simulink model "single_phase_grid_connected_inverter"  (R2022b)
settings: Solver=FixedStepDiscrete  StartTime=0.0  StopTime=0.5  FixedStep=1e-6  RelTol=1e-3
libraries: spsSeriesRLCBranchLib x9, spsFourierLib x8, spsMosfetLib x4, spsCurrentMeasurementLib x3, simulink x3, spsVoltageMeasurementLib x3, spsMeanLib x2, spsRMSLib x2, spsDCVoltageSourceLib x1, spsIdealSwitchLib x1, spspowerguiLib x1, spsControlledVoltageSourceLib x1
(part 2 of 2)

== matlab function single_phase_grid_connected_inverter/MATLAB Function20 ==
  data: u_alpha input; theta output; u_beta input; qerror output
function [theta, qerror] = SRF_PLL(u_alpha, u_beta)
% 同步旋转坐标系锁相环 SRF-PLL
% 【已修改为：纯自适应频率版本 → 和你主循环PLL完全一致】
% 输入：u_alpha, u_beta
% 输出：theta 锁相相位, qerror q分量（趋近0）

    %% ===================== 1. 固定参数 =====================
    Ts = 5e-5;               % 20kHz 采样步长（必须匹配）
    
    % PI参数（和你主循环一致）
    kp_pll = 200;
    ki_pll = 7000;

    %% ===================== 2. 持久变量 =====================
    persistent theta_prev
    persistent integral_pll
    
    if isempty(theta_prev)
        theta_prev = 0;
        integral_pll = 0;
    end

    %% ===================== 3. Park 变换 =====================
    cos_theta = cos(theta_prev);
    sin_theta = sin(theta_prev);
    
    u_d =  u_alpha * cos_theta + u_beta * sin_theta;
    u_q = -u_alpha * sin_theta + u_beta * cos_theta;
    
    qerror = u_q;  % q分量（锁相成功→0）

    %% ===================== 4. PI控制器（我的版本：直接输出ω） =====================
    integral_pll = integral_pll + qerror * Ts;          % 积分
    omega_pll    = kp_pll * qerror + ki_pll * integral_pll; % 直接输出角频率

    %% ===================== 5. 积分生成相位 =====================
    theta = theta_prev + omega_pll * Ts;

    %% ===================== 6. 相位归一化（±π） =====================
    if theta > pi
        theta = theta - 2*pi;
    elseif theta < -pi
        theta = theta + 2*pi;
    end

    %% ===================== 7. 更新状态 =====================
    theta_prev = theta;
end

== matlab function single_phase_grid_connected_inverter/级联谐波抑制4 ==
  data: u input; y output
function y = Cascade_Notch_Filter(u)
% 级联陷波滤波器：滤除3/5/7次固定频率谐波（150/250/350Hz）
% 输入u：待滤波的标量信号
% 输出y：滤波后的标量信号
% 适配：20kHz采样率（Ts=5e-5），和你的控制环完全对齐

    persistent x3_1 x3_2 x5_1 x5_2 x7_1 x7_2 first_run
    persistent b3_0 b3_1 b3_2 a3_1 a3_2
    persistent b5_0 b5_1 b5_2 a5_1 a5_2
    persistent b7_0 b7_1 b7_2 a7_1 a7_2

    %% ===================== 1. 初始化：仅首次运行 =====================
    if isempty(first_run)
        % --- 固定参数 ---
        Fs = 2e4;          % 采样频率 20kHz
        Ts = 1/Fs;            % 采样周期 5e-5s
        wc = 10;              % 截止角频率 25 rad/s
        
        % 目标谐波频率
        w3 = 2*pi*150;  % 3次谐波 150Hz
        w5 = 2*pi*250;  % 5次谐波 250Hz
        w7 = 2*pi*350;  % 7次谐波 350Hz

        % --- Tustin变换预计算系数 ---
        k = 2/Ts;
        k2 = k*k;

        % --- 3次滤波器系数 ---
        [b3_0, b3_1, b3_2, a3_1, a3_2] = calc_coeff(w3, wc, k, k2);
        % --- 5次滤波器系数 ---
        [b5_0, b5_1, b5_2, a5_1, a5_2] = calc_coeff(w5, wc, k, k2);
        % --- 7次滤波器系数 ---
        [b7_0, b7_1, b7_2, a7_1, a7_2] = calc_coeff(w7, wc, k, k2);

        % --- 显式初始化状态变量为标量 ---
        x3_1 = 0; x3_2 = 0;
        x5_1 = 0; x5_2 = 0;
        x7_1 = 0; x7_2 = 0;
        
        first_run = 1;
    end

    %% ===================== 2. 级联滤波计算（显式差分方程） =====================
    % --- 第1级：3次谐波滤波 ---
    y3 = b3_0*u + x3_1;
    x3_1_next = b3_1*u - a3_1*y3 + x3_2;
    x3_2_next = b3_2*u - a3_2*y3;
    
    % --- 第2级：5次谐波滤波 ---
    y5 = b5_0*y3 + x5_1;
    x5_1_next = b5_1*y3 - a5_1*y5 + x5_2;
    x5_2_next = b5_2*y3 - a5_2*y5;
    
    % --- 第3级：7次谐波滤波 ---
    y7 = b7_0*y5 + x7_1;
    x7_1_next = b7_1*y5 - a7_1*y7 + x7_2;
    x7_2_next = b7_2*y5 - a7_2*y7;
    
    % --- 更新状态变量 ---
    x3_1 = x3_1_next; x3_2 = x3_2_next;
    x5_1 = x5_1_next; x5_2 = x5_2_next;
    x7_1 = x7_1_next; x7_2 = x7_2_next;
    
    % --- 最终输出 ---
    y = y7;

end

%% ===================== 局部函数：预计算滤波器系数 =====================
function [b0, b1, b2, a1, a2] = calc_coeff(wn, wc, k, k2)
    % 连续域：G(s) = (s^2 + wn^2) / (s^2 + 2*wc*s + wn^2)
    % Tustin离散化：s = k*(z-1)/(z+1)
    
    % 连续域系数
    num_b0 = 1; num_b1 = 0; num_b2 = wn^2;
    den_a0 = 1; den_a1 = 2*wc; den_a2 = wn^2;
    
    % 离散化计算
    B0 = num_b0*k2 + num_b1*k + num_b2;
    B1 = 2*num_b2 - 2*num_b0*k2;
    B2 = num_b0*k2 - num_b1*k + num_b2;
    
    A0 = den_a0*k2 + den_a1*k + den_a2;
    A1 = 2*den_a2 - 2*den_a0*k2;
    A2 = den_a0*k2 - den_a1*k + den_a2;
    
    % 归一化（a0=1）
    b0 = B0 / A0;
    b1 = B1 / A0;
    b2 = B2 / A0;
    a1 = A1 / A0;
    a2 = A2 / A0;
end

== matlab function single_phase_grid_connected_inverter/MATLAB Function11 ==
  data: u_alpha input; theta output; u_beta input; qerror output
function [theta, qerror] = SRF_PLL(u_alpha, u_beta)
% 同步旋转坐标系锁相环 SRF-PLL（严格匹配框图逻辑）
% 输入
%   u_alpha:  α轴输入信号（对应框图的v'，与电网电压同相）
%   u_beta:   β轴输入信号（对应框图的qv'，与电网电压正交90°）
% 输出
%   theta:    锁相得到的电网相位 [0, 2π)
%   qerror:   q轴相位误差（锁相锁定时趋近于0）
% 适配：仿真步长 Ts=1e-5（10kHz采样），基波频率50Hz

    %% ===================== 1. 固定参数配置 =====================
    Ts = 1e-5;               % 采样时间，必须与全局仿真步长完全一致
    f0 = 50;                  % 电网额定基波频率 (Hz)
    w0 = 2 * pi * f0;        % 额定角频率 (rad/s)
    
    % PI控制器参数（适配10kHz采样，可按需调整）
    kp_pll = 60;              % 比例系数：增大加快锁相响应，过大易振荡
    ki_pll = 5000;            % 积分系数：增大减小稳态相位误差，过大影响稳定性

    %% ===================== 2. 持久变量初始化（仅首次运行执行） =====================
    persistent theta_prev     % 上一拍的锁相相位
    persistent xi_pll         % PI控制器的积分项（抗饱和）
    
    if isempty(theta_prev)
        theta_prev = 0;       % 相位初始值清零
        xi_pll = 0;           % 积分项初始值清零
    end

    %% ===================== 3. αβ/dq 帕克变换（核心鉴相环节） =====================
    % 标准帕克变换矩阵，严格匹配框图逻辑
    % [u_d]   = [ cosθ   sinθ ] [u_alpha]
    % [u_q]     [ -sinθ  cosθ ] [u_beta ]
    cos_theta = cos(theta_prev);
    sin_theta = sin(theta_prev);
    
    u_d = u_alpha * cos_theta + u_beta * sin_theta;  % d轴分量（对应电压幅值）
    u_q = -u_alpha * sin_theta + u_beta * cos_theta; % q轴分量（相位误差）
    
    qerror = u_q; % 输出q轴相位误差，锁相锁定时qerror→0

    %% ===================== 4. PI环路控制器 =====================
    % 位置式PI控制器，带积分抗饱和
    xi_pll = xi_pll + ki_pll * Ts * qerror;  % 积分项更新
    delta_w = kp_pll * qerror + xi_pll;      % 频率偏差量
    w_pll = w0 + delta_w;                     % 锁相得到的实时角频率

    %% ===================== 5. 积分环节（1/s）生成相位 =====================
    % 前向欧拉离散化，对应框图的1/s积分环节
    theta = theta_prev + Ts * w_pll;
    
    % 相位归一化到 [0, 2π)，防止数值溢出
    theta = mod(theta, 2 * pi);

    %% ===================== 6. 更新状态变量（为下一拍迭代准备） =====================
    theta_prev = theta;

end

== matlab function single_phase_grid_connected_inverter/MATLAB Function2 ==
  data: u input; y output
function y = SecondOrderPadeDelay_1p5Ts(u)
% 二阶Padé逼近1.5Ts延迟模块（直接从闭环仿真提取，已验证直流增益=1）
% 输入：u - 待延迟的信号（如PR控制器输出）
% 输出：y - 延迟后的信号
% 适配：与你的闭环仿真参数100%匹配，直流增益严格等于1

persistent u_prev1 u_prev2 y_prev1 y_prev2 first_run

%% 初始化：仅首次运行
if isempty(first_run)
    % 初始化状态变量（二阶需要2个历史输入+2个历史输出）
    u_prev1 = 0;
    u_prev2 = 0;
    y_prev1 = 0;
    y_prev2 = 0;
    
    first_run = true;
end

%% 【核心】直接从闭环仿真提取的系数（已验证直流增益=1）
b0 = 0.076923076923077;
b1 = 0.153846153846154;
b2 = 1.000000000000000;
a1 = -0.153846153846154;
a2 = -0.076923076923077;

%% 二阶离散差分方程计算延迟输出
y = b0*u + b1*u_prev1 + b2*u_prev2 ...
    + a1*y_prev1 + a2*y_prev2;

%% 更新状态变量（供下一时刻使用）
u_prev2 = u_prev1;
u_prev1 = u;
y_prev2 = y_prev1;
y_prev1 = y;
end

== matlab function single_phase_grid_connected_inverter/MATLAB Function3 ==
  settings: updateMethod=DISCRETE
  data: u input; y output
function y = PR_Controller(u)
% 准谐振PR控制器，和你的.m文件1:1完全匹配
% 输入u：误差信号 error = Iref - iL2
% 输出y：PR控制器输出的调制波

persistent x_prev1 x_prev2 y_prev1 y_prev2 first_run

%% 1. 固定参数（和.m文件完全一致，无任何修改）
Ts = 5e-5;           % 采样时间 (s)，20kHz控制环
Kp = 0.254;          % PR比例系数
Kr = 50;             % PR谐振系数
w0 = 2*pi*50;        % 基波角频率 (50Hz)，和.m文件写法完全对齐
wi = pi;             % PR谐振带宽

%% 2. 初始化状态变量（仅首次运行，和.m文件初始值一致）
if isempty(first_run)
    x_prev1 = 0;  % 对应.m文件的x1_pr：上一时刻的误差
    x_prev2 = 0;  % 对应.m文件的x2_pr：上两时刻的误差
    y_prev1 = 0;  % 对应.m文件的y1_pr：上一时刻的输出
    y_prev2 = 0;  % 对应.m文件的y2_pr：上两时刻的输出
    first_run = true;
end

%% 3. 离散化系数计算（和.m文件公式、参数完全一致）
a0_pr = 4 + 2*wi*Ts + w0^2*Ts^2;
a1_pr = 2*w0^2*Ts^2 - 8;
a2_pr = 4 - 2*wi*Ts + w0^2*Ts^2;

b0_pr = 4*Kp + 4*Kp*wi*Ts + 4*Kr*wi*Ts + Kp*w0^2*Ts^2;
b1_pr = 2*Kp*w0^2*Ts^2 - 8*Kp;
b2_pr = 4*Kp - 4*Kp*wi*Ts - 4*Kr*wi*Ts + Kp*w0^2*Ts^2;

%% 4. 差分方程计算输出（和.m文件公式完全一致，符号无错误）
y = (b0_pr*u + b1_pr*x_prev1 + b2_pr*x_prev2 ...
    - a1_pr*y_prev1 - a2_pr*y_prev2) / a0_pr;

%% 5. 输出限幅（和.m文件完全一致，[-1,1]）
MODULATION_MAX = 1;
MODULATION_MIN = -1;
y = max(min(y, MODULATION_MAX), MODULATION_MIN);

%% 6. 更新状态变量（和.m文件执行顺序完全一致：先算输出→再限幅→最后更新）
x_prev2 = x_prev1;
x_prev1 = u;
y_prev2 = y_prev1;
y_prev1 = y;

end

== matlab function single_phase_grid_connected_inverter/MATLAB Function6 ==
  data: alpha input; d output; beta input; theta input; q output
function [d, q] = Park_Transform(alpha, beta, theta)
% Park变换模块（直接输入SOGI-FLL的theta，无内部积分）
% 输入：
%   alpha - α轴分量（SOGI-FLL的U_prime）
%   beta  - β轴分量（SOGI-FLL的deltaU_prime）
%   theta - 瞬时相位（SOGI-FLL直接输出的theta）
% 输出：
%   d         - d轴（直轴）分量
%   q         - q轴（交轴）分量
%   cos_theta - 相位θ的余弦值（新增输出）
%   sin_theta - 相位θ的正弦值（新增输出）

%% 核心计算
cos_theta = cos(theta);  % 相位θ的余弦值
sin_theta = sin(theta);  % 相位θ的正弦值


% 修正后的 Park 变换公式（d轴对齐同相分量 beta）
d =  alpha * cos_theta + beta * sin_theta;
q = -alpha * sin_theta + beta * cos_theta;
end

== matlab function single_phase_grid_connected_inverter/1.5倍延时 ==
  data: u input; y output
function y = SecondOrderPadeDelay_1p5Ts(u)
% 二阶Padé逼近1.5Ts延迟模块（直接从闭环仿真提取，已验证直流增益=1）
% 输入：u - 待延迟的信号（如PR控制器输出）
% 输出：y - 延迟后的信号
% 适配：与你的闭环仿真参数100%匹配，直流增益严格等于1

persistent u_prev1 u_prev2 y_prev1 y_prev2 first_run

%% 初始化：仅首次运行
if isempty(first_run)
    % 初始化状态变量（二阶需要2个历史输入+2个历史输出）
    u_prev1 = 0;
    u_prev2 = 0;
    y_prev1 = 0;
    y_prev2 = 0;
    
    first_run = true;
end

%% 【核心】直接从闭环仿真提取的系数（已验证直流增益=1）
b0 = 0.076923076923077;
b1 = 0.153846153846154;
b2 = 1.000000000000000;
a1 = -0.153846153846154;
a2 = -0.076923076923077;

%% 二阶离散差分方程计算延迟输出
y = b0*u + b1*u_prev1 + b2*u_prev2 ...
    + a1*y_prev1 + a2*y_prev2;

%% 更新状态变量（供下一时刻使用）
u_prev2 = u_prev1;
u_prev1 = u;
y_prev2 = y_prev1;
y_prev1 = y;
end

== matlab function single_phase_grid_connected_inverter/MATLAB Function7 ==
  settings: updateMethod=DISCRETE
  data: U_in input; U_prime output; deltaU_prime output
function [U_prime, deltaU_prime] = SOGI_FLL_Process(U_in)
% SOGI-FLL for Simulink: 逐点更新，内置相位积分，维护状态记忆
% 输入：U_in   - 当前时刻输入电压（标量）
% 输出：U_prime      - α轴同相输出（标量）
%       deltaU_prime - β轴正交输出（标量）
%       omega0       - 当前角频率（rad/s，标量）
%       theta        - 积分得到的瞬时相位（rad，标量，θ=∫ωdt）

%% 固定参数
dt = 1e-5;               % 仿真步长，必须与Simulink求解器步长一致
K = 1.414;               % SOGI增益
K1 = 0.25;               % 直流消除器增益
gamma = 20;              % FLL增益（你已调至46，加快收敛）
omega0_init = 100*pi;    % 初始角频率（50Hz）
w_max = 2*pi*60;         % 频率上限（60Hz）
w_min = 2*pi*40;         % 频率下限（40Hz）

%% 状态变量持久化（Simulink中必须用persistent）
persistent x1_prev x2_prev x3_prev omega0_prev theta_prev first_run

if isempty(first_run)
    % 首次运行初始化
    x1_prev = 0;
    x2_prev = 0;
    x3_prev = 0;
    omega0_prev = omega0_init;
    theta_prev = 0;       % 相位积分初始值（θ₀=0，匹配输入无初相）
    first_run = false;
end

%% 1. 计算状态导数（逐点，无矩阵）
A11 = -K1 * omega0_prev; A12 = -K1 * omega0_prev; A13 = 0;
A21 = -K  * omega0_prev; A22 = -K  * omega0_prev; A23 = -omega0_prev^2;
A31 = 0;                  A32 = 1;                   A33 = 0;

B1 = K1 * omega0_prev;
B2 = K  * omega0_prev;
B3 = 0;

dx1dt = A11*x1_prev + A12*x2_prev + A13*x3_prev + B1*U_in;
dx2dt = A21*x1_prev + A22*x2_prev + A23*x3_prev + B2*U_in;
dx3dt = A31*x1_prev + A32*x2_prev + A33*x3_prev + B3*U_in;

%% 2. 前向欧拉更新状态
x1_curr = x1_prev + dt * dx1dt;
x2_curr = x2_prev + dt * dx2dt;
x3_curr = x3_prev + dt * dx3dt;

%% 3. FLL频率更新
deltaU = U_in - x1_curr - x2_curr;
deltaU_prime_k = omega0_prev * x3_curr;
epsilon_f = deltaU * deltaU_prime_k;
domega0dt = -gamma * epsilon_f;
omega0_curr = omega0_prev + dt * domega0dt;

% 频率限幅
omega0_curr = max(min(omega0_curr, w_max), w_min);

%% 4. 内置相位积分（梯形积分，精度更高）
% 梯形积分：theta = theta_prev + (当前ω + 前一时刻ω) * dt / 2
theta_curr = theta_prev + (omega0_curr + omega0_prev) * dt / 2;
% 相位归一化（限制在[-π, π]，避免数值溢出）
theta_curr = mod(theta_curr + pi, 2*pi) - pi;

%% 5. 输出
U_prime = x2_curr;
deltaU_prime = omega0_prev * x3_curr;  % 用前一时刻ω₀计算正交分量
omega0 = omega0_curr;
theta = theta_curr;  % 新增相位输出

%% 6. 更新状态，供下一时刻使用
x1_prev = x1_curr;
x2_prev = x2_curr;
x3_prev = x3_curr;
omega0_prev = omega0_curr;
theta_prev = theta_curr;  % 更新相位状态
end

== matlab function single_phase_grid_connected_inverter/MATLAB Function4 ==
  settings: updateMethod=DISCRETE
  data: u input; y output
function y = PR_Controller(u)
% 准谐振PR控制器，和你的.m文件1:1完全匹配
% 输入u：误差信号 error = Iref - iL2
% 输出y：PR控制器输出的调制波

persistent x_prev1 x_prev2 y_prev1 y_prev2 first_run

%% 1. 固定参数（和.m文件完全一致，无任何修改）
Ts = 5e-5;           % 采样时间 (s)，20kHz控制环
Kp = 0.2;               % PR比例系数
Kr = 40.92;             % PR谐振系数
w0 = 2*pi*50;        % 基波角频率 (50Hz)，和.m文件写法完全对齐
wi = pi;             % PR谐振带宽

%% 2. 初始化状态变量（仅首次运行，和.m文件初始值一致）
if isempty(first_run)
    x_prev1 = 0;  % 对应.m文件的x1_pr：上一时刻的误差
    x_prev2 = 0;  % 对应.m文件的x2_pr：上两时刻的误差
    y_prev1 = 0;  % 对应.m文件的y1_pr：上一时刻的输出
    y_prev2 = 0;  % 对应.m文件的y2_pr：上两时刻的输出
    first_run = true;
end

%% 3. 离散化系数计算（和.m文件公式、参数完全一致）
a0_pr = 4 + 2*wi*Ts + w0^2*Ts^2;
a1_pr = 2*w0^2*Ts^2 - 8;
a2_pr = 4 - 2*wi*Ts + w0^2*Ts^2;

b0_pr = 4*Kp + 4*Kp*wi*Ts + 4*Kr*wi*Ts + Kp*w0^2*Ts^2;
b1_pr = 2*Kp*w0^2*Ts^2 - 8*Kp;
b2_pr = 4*Kp - 4*Kp*wi*Ts - 4*Kr*wi*Ts + Kp*w0^2*Ts^2;

%% 4. 差分方程计算输出（和.m文件公式完全一致，符号无错误）
y = (b0_pr*u + b1_pr*x_prev1 + b2_pr*x_prev2 ...
    - a1_pr*y_prev1 - a2_pr*y_prev2) / a0_pr;

%% 5. 输出限幅（和.m文件完全一致，[-1,1]）
MODULATION_MAX = 1;
MODULATION_MIN = -1;
y = max(min(y, MODULATION_MAX), MODULATION_MIN);

%% 6. 更新状态变量（和.m文件执行顺序完全一致：先算输出→再限幅→最后更新）
x_prev2 = x_prev1;
x_prev1 = u;
y_prev2 = y_prev1;
y_prev1 = y;

end

== matlab function single_phase_grid_connected_inverter/MATLAB Function5 ==
  data: alpha input; d output; beta input; theta input; q output
function [d, q] = Park_Transform(alpha, beta, theta)
% Park变换模块（直接输入SOGI-FLL的theta，无内部积分）
% 输入：
%   alpha - α轴分量（SOGI-FLL的U_prime）
%   beta  - β轴分量（SOGI-FLL的deltaU_prime）
%   theta - 瞬时相位（SOGI-FLL直接输出的theta）
% 输出：
%   d         - d轴（直轴）分量
%   q         - q轴（交轴）分量
%   cos_theta - 相位θ的余弦值（新增输出）
%   sin_theta - 相位θ的正弦值（新增输出）

%% 核心计算
cos_theta = cos(theta);  % 相位θ的余弦值
sin_theta = sin(theta);  % 相位θ的正弦值


% 修正后的 Park 变换公式（d轴对齐同相分量 beta）
d =  alpha * cos_theta + beta * sin_theta;
q = -alpha * sin_theta + beta * cos_theta;
end

== matlab function single_phase_grid_connected_inverter/MATLAB Function8 ==
  settings: updateMethod=DISCRETE
  data: U_in input; U_prime output; deltaU_prime output
function [U_prime, deltaU_prime] = SOGI_FLL_Process(U_in)
% SOGI-FLL for Simulink: 逐点更新，内置相位积分，维护状态记忆
% 输入：U_in   - 当前时刻输入电压（标量）
% 输出：U_prime      - α轴同相输出（标量）
%       deltaU_prime - β轴正交输出（标量）
%       omega0       - 当前角频率（rad/s，标量）
%       theta        - 积分得到的瞬时相位（rad，标量，θ=∫ωdt）

%% 固定参数
dt = 1e-5;               % 仿真步长，必须与Simulink求解器步长一致
K = 1.414;               % SOGI增益
K1 = 0.25;               % 直流消除器增益
gamma = 20;              % FLL增益（你已调至46，加快收敛）
omega0_init = 100*pi;    % 初始角频率（50Hz）
w_max = 2*pi*60;         % 频率上限（60Hz）
w_min = 2*pi*40;         % 频率下限（40Hz）

%% 状态变量持久化（Simulink中必须用persistent）
persistent x1_prev x2_prev x3_prev omega0_prev theta_prev first_run

if isempty(first_run)
    % 首次运行初始化
    x1_prev = 0;
    x2_prev = 0;
    x3_prev = 0;
    omega0_prev = omega0_init;
    theta_prev = 0;       % 相位积分初始值（θ₀=0，匹配输入无初相）
    first_run = false;
end

%% 1. 计算状态导数（逐点，无矩阵）
A11 = -K1 * omega0_prev; A12 = -K1 * omega0_prev; A13 = 0;
A21 = -K  * omega0_prev; A22 = -K  * omega0_prev; A23 = -omega0_prev^2;
A31 = 0;                  A32 = 1;                   A33 = 0;

B1 = K1 * omega0_prev;
B2 = K  * omega0_prev;
B3 = 0;

dx1dt = A11*x1_prev + A12*x2_prev + A13*x3_prev + B1*U_in;
dx2dt = A21*x1_prev + A22*x2_prev + A23*x3_prev + B2*U_in;
dx3dt = A31*x1_prev + A32*x2_prev + A33*x3_prev + B3*U_in;

%% 2. 前向欧拉更新状态
x1_curr = x1_prev + dt * dx1dt;
x2_curr = x2_prev + dt * dx2dt;
x3_curr = x3_prev + dt * dx3dt;

%% 3. FLL频率更新
deltaU = U_in - x1_curr - x2_curr;
deltaU_prime_k = omega0_prev * x3_curr;
epsilon_f = deltaU * deltaU_prime_k;
domega0dt = -gamma * epsilon_f;
omega0_curr = omega0_prev + dt * domega0dt;

% 频率限幅
omega0_curr = max(min(omega0_curr, w_max), w_min);

%% 4. 内置相位积分（梯形积分，精度更高）
% 梯形积分：theta = theta_prev + (当前ω + 前一时刻ω) * dt / 2
theta_curr = theta_prev + (omega0_curr + omega0_prev) * dt / 2;
% 相位归一化（限制在[-π, π]，避免数值溢出）
theta_curr = mod(theta_curr + pi, 2*pi) - pi;

%% 5. 输出
U_prime = x2_curr;
deltaU_prime = omega0_prev * x3_curr;  % 用前一时刻ω₀计算正交分量
omega0 = omega0_curr;
theta = theta_curr;  % 新增相位输出

%% 6. 更新状态，供下一时刻使用
x1_prev = x1_curr;
x2_prev = x2_curr;
x3_prev = x3_curr;
omega0_prev = omega0_curr;
theta_prev = theta_curr;  % 更新相位状态
end
